simulink model "arm_trajectory"  (R2025b)
settings: Solver=ode45  StartTime=0.0  StopTime=20  MaxStep=0.05  RelTol=1e-3
settings Model: Creator=Krishang  LastModifiedBy=Krishang

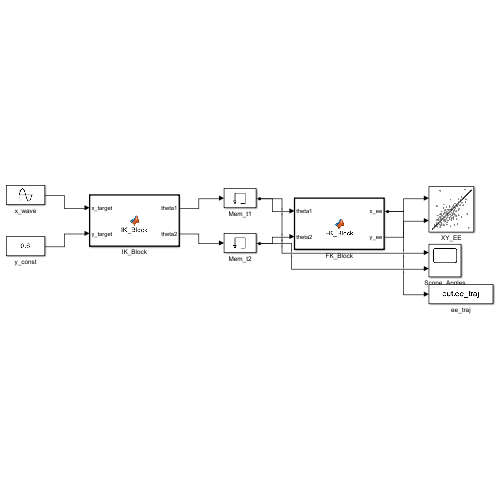
[thumbnail: Simulink's stored preview of the top-level diagram]
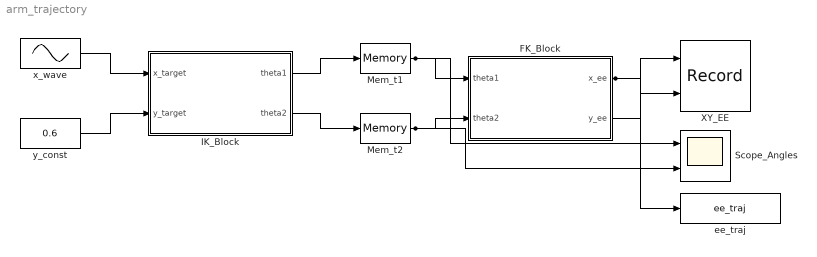
== system arm_trajectory ==
  FK_Block : MATLAB Function  TreatAsAtomicUnit=on
  IK_Block : MATLAB Function  TreatAsAtomicUnit=on
  Mem_t1 : Memory
  Mem_t2 : Memory
  Scope_Angles : Scope  NumInputPorts=2
  XY_EE : Record  NumPorts=2.0  FileSettingsInternal="{\"entries\":[{\"content\":{\"excelSettings\":{\"content\":{},\"type\":\"Streamout.ExcelSettings\"},\"parquetSettings\":{\"content\":{},\"type\":\"Streamout.ParquetSettings\"}},\"type\":\"Streamout.FileSettingStorage\",\"uuid\":\"\"}],\"packageUris\":[\"http:\\/\\/schema.mathworks.com\\/mf0\\/streamout_blocks\\/R2020a\"],\"version\":\"1.0\"}"  FrameSettings=[0, 0]  Layout=[1 1]  SignalsInternal="{\"entries\":[{\"content\":{\"signals\":[{\"content\":{\"blockPath\":[],\"dimensions\":[1],\"domain\":\"\",\"lineColor\":\"#a2142f\",\"plots\":[ 1 ],\"port\":1,\"signalID\":1,\"signalName\":\"XY Graph:1\"},\"type\":\"RecordBlkView.Signal\",\"uuid\":\"\"},{\"content\":{\"blockPath\":[],\"dimensions\":[1],\"domain\":\"\",\"lineColor\":\"#139fff\",\"plots\":[ 1 ],\"port\":2,\"signalID\":2,\"signalName\":\"XY Graph:2\"},\"type\":\"RecordBlkView.Signal\",\"uuid\":\"\"}]},\"type\":\"RecordBlkView.InputSignals\",\"uuid\":\"\"}],\"packageUris\":[\"http:\\/\\/schema.mathworks.com\\/mf0\\/streamout_blocks\\/R2020a\"],\"version\":\"1.0\"}"  VisualizationBindings="{\"xyplotplugin\":{\"info\":[{\"series\":[{\"bindingParametersList\":[{\"parameter\":\"X-Axis\",\"signalID\":1,\"signalName\":\"XY Graph:1\"},{\"parameter\":\"Y-Axis\",\"signalID\":2,\"signalName\":\"XY Graph:2\"}],\"seriesID\":0}],\"subplotID\":1}]}}"  CompatibilityTag=XY
  ee_traj : ToWorkspace  VariableName=ee_traj  SampleTime=-1
  x_wave : Sin  Amplitude=0.4  Bias=1.0  Frequency=0.5  SampleTime=0
  y_const : Constant  Value=0.6
  wires:
  x_wave/1 -> IK_Block/1(x_target)
  y_const/1 -> IK_Block/2(y_target)
  IK_Block/1(theta1) -> Mem_t1/1
  IK_Block/2(theta2) -> Mem_t2/1
  Mem_t1/1 -> FK_Block/1(theta1), Scope_Angles/1
  Mem_t2/1 -> FK_Block/2(theta2), Scope_Angles/2
  FK_Block/1(x_ee) -> XY_EE/1, ee_traj/1
  FK_Block/2(y_ee) -> XY_EE/2

== matlab function arm_trajectory/IK_Block ==
  data: x_target input; theta1 output; y_target input; theta2 output
function [theta1, theta2] = IK_Block(x_target, y_target)
L1 = 1.0; L2 = 0.8;
r     = sqrt(x_target^2 + y_target^2);
r_max = L1 + L2;
r_min = abs(L1 - L2);
r_s   = max(r_min + 1e-6, min(r_max - 1e-6, r));
if r > 1e-9
    xs = x_target * (r_s / r);
    ys = y_target * (r_s / r);
else
    xs = r_s; ys = 0;
end
c2     = max(-1, min(1, (xs^2 + ys^2 - L1^2 - L2^2) / (2*L1*L2)));
theta2 = atan2(sqrt(1 - c2^2), c2);
alpha  = atan2(ys, xs);
beta   = atan2(L2*sin(theta2), L1 + L2*cos(theta2));
theta1 = atan2(sin(alpha - beta), cos(alpha - beta));
end

== matlab function arm_trajectory/FK_Block ==
  data: theta1 input; x_ee output; theta2 input; y_ee output
function [x_ee, y_ee] = FK_Block(theta1, theta2)
L1 = 1.0; L2 = 0.8;
x_ee = L1*cos(theta1) + L2*cos(theta1 + theta2);
y_ee = L1*sin(theta1) + L2*sin(theta1 + theta2);
end
